simulink model "Controlador_PID_de_movimiento_discreto"  (R2023b)
settings: Solver=VariableStepAuto  StartTime=0.0  StopTime=14  RelTol=1e-3
values from neighbouring files (symbols this model uses):
  alpha_Cu = 3.9e-3    (= 0.0039)    [definicio_cte.m]
  b_a = 0.0396    [definicio_cte.m]
  b_eq = b_m + b_l/(r^2)    (= 1.98611111111e-05)    [definicio_cte.m]
  C_ts = 0.818    [definicio_cte.m]
  g = 9.80665    [definicio_cte.m]
  J_eq = J_m + J_l/(r^2)    (= 1.97847222222e-05)    [definicio_cte.m]
  k_l = m*l_cm + m_l*l_l    (= 0.25)    [definicio_cte.m]
  K_omega_2 = 3.0720e7    (= 30720000)    [definicio_cte.m]
  K_sa = 31.656    [definicio_cte.m]
  K_theta_2 = 9600    [definicio_cte.m]
  K_theta_i = 3.2768e10    (= 32768000000)    [definicio_cte.m]
  L_d = 6.6e-3    (= 0.0066)    [definicio_cte.m]
  L_ls = 0.8e-3    (= 0.0008)    [definicio_cte.m]
  L_q = 5.8e-3    (= 0.0058)    [definicio_cte.m]
  lambda_m = 0.016    [definicio_cte.m]
  lim_inf = -sqrt(2) * 48 / sqrt(3)    [definicio_cte.m]
  lim_sup = sqrt(2) * 48 / sqrt(3)    [definicio_cte.m]
  P_p = 3    [definicio_cte.m]
  r = 120    [definicio_cte.m]
  R_0 = 5000 * L_ls    (= 4)    [definicio_cte.m]
  R_d = 5000 * L_d    (= 33)    [definicio_cte.m]
  R_q = 5000 * L_q    (= 29)    [definicio_cte.m]
  R_sREF = 1.02    [definicio_cte.m]
  R_tsamb = 146.7    [definicio_cte.m]
  T_amb = 25    [definicio_cte.m]
  T_sREF = 20    [definicio_cte.m]
  tau = 20    [definicio_cte.m]
  Ts = 1.256e-4    (= 0.0001256)    [definicio_cte.m]
  w_modul = 6000*4    (= 24000)    [definicio_cte.m]
  wn_i = 6000*3    (= 18000)    [definicio_cte.m]
  wn_theta = 2000*3    (= 6000)    [definicio_cte.m]
  xita_i = 1    [definicio_cte.m]
  xita_modul = 1    [definicio_cte.m]
  xita_theta = 1    [definicio_cte.m]
undefined symbols (not defined in the file or in its folder): K_sia, magnitude
libraries: simulink x16
(part 1 of 2)
settings Model: Creator=MSI  LastModifiedBy=MSI

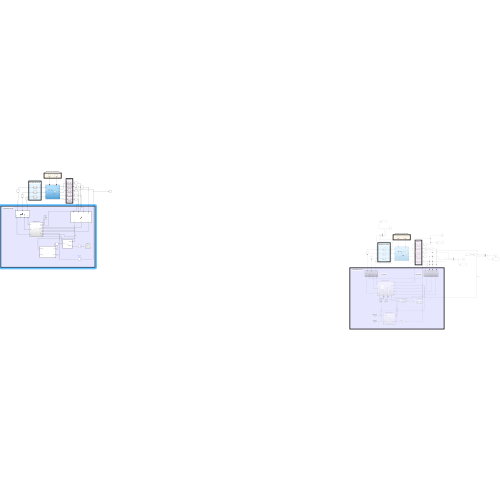
[thumbnail: Simulink's stored preview of the top-level diagram]
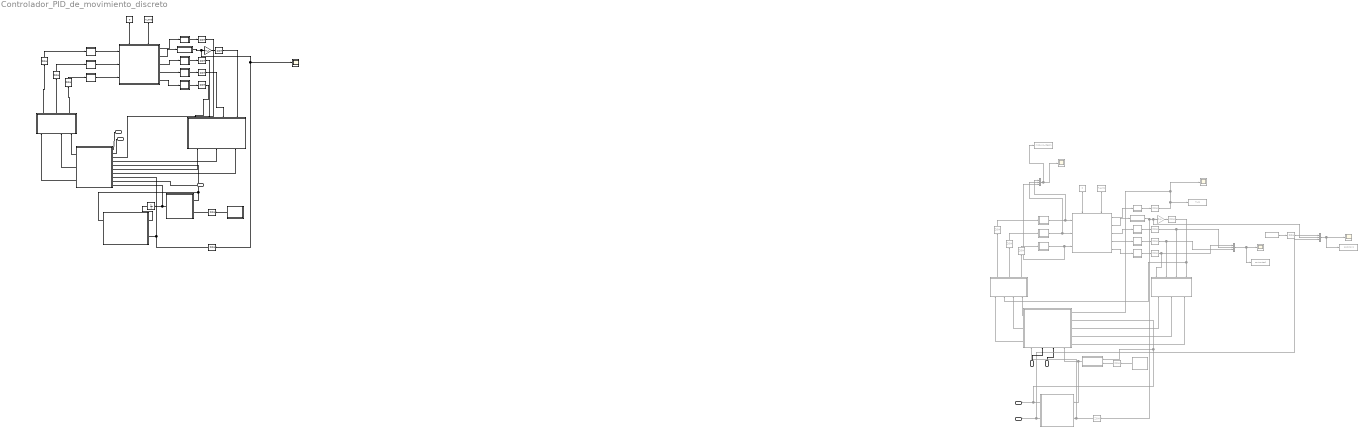
== system Controlador_PID_de_movimiento_discreto ==
  note: Controlador Parcial
  note: Sensores
  note: Entradas de perturbación
  note: Modulador de Tensión
  note: Modulador de Tensión
  note: Controlador Parcial
  note: T.P Directa
  note: Sensores
  note: Entradas de perturbación
  note: T.P Inversa
  i0s_ref : Inport
  ids_ref : Inport  Port=2
  g : Inport  Port=3
  ids*1 : Inport  Port=4
  i0s*1 : Inport  Port=5
  . : Subsystem
      settings: PortSchema="{\"entries\":[{\"content\":{\"sides\":[{\"content\":{\"connectorIds\":[\"In1\",\"In2\",\"In3\"]},\"type\":\"ConnectorPlacement.EquallySpacedRectSide\",\"uuid\":\"a2221977-a2db-4f9f-a6b6-e4e93ab83132\"},{\"content\":{\"connectorIds\":[\"Out1\",\"Out2\",\"Out3\",\"Out4\",\"Out5\"],\"side\":\"RIGHT\"},\"type\":\"ConnectorPlacement.EquallySpacedRectSide\",\"uuid\":\"4d1b64fb-cd5f-444c-9c55-dd968f667727\"},{\"content\":{\"connectorIds\":[\"In4\",\"In5\"],\"side\":\"TOP\"},\"type\":\"ConnectorPlacement.EquallySpacedRectSide\",\"uuid\":\"feec2d7e-2013-4827-9d2d-5413e6a364ce\"},{\"content\":{\"side\":\"BOTTOM\"},\"type\":\"ConnectorPlacement.EquallySpacedRectSide\",\"uuid\":\"a4e68a75-7272-4a37-88ea-97e0fe693470\"}]},\"type\":\"ConnectorPlacement.EquallySpacedConnector\",\"uuid\":\"3fef7616-1be8-4199-84fe-e5c97ae42ef2\"}],\"packageUris\":[\"http://schema.mathworks.com/mf0/Connector/R2020b\"],\"version\":\"1.0\"}"
  .1 : Subsystem  Commented=on
      settings: PortSchema="{\"entries\":[{\"content\":{\"sides\":[{\"content\":{\"connectorIds\":[\"In1\",\"In2\",\"In3\"]},\"type\":\"ConnectorPlacement.EquallySpacedRectSide\",\"uuid\":\"a2221977-a2db-4f9f-a6b6-e4e93ab83132\"},{\"content\":{\"connectorIds\":[\"Out1\",\"Out2\",\"Out3\",\"Out4\",\"Out5\"],\"side\":\"RIGHT\"},\"type\":\"ConnectorPlacement.EquallySpacedRectSide\",\"uuid\":\"4d1b64fb-cd5f-444c-9c55-dd968f667727\"},{\"content\":{\"connectorIds\":[\"In4\",\"In5\"],\"side\":\"TOP\"},\"type\":\"ConnectorPlacement.EquallySpacedRectSide\",\"uuid\":\"feec2d7e-2013-4827-9d2d-5413e6a364ce\"},{\"content\":{\"side\":\"BOTTOM\"},\"type\":\"ConnectorPlacement.EquallySpacedRectSide\",\"uuid\":\"a4e68a75-7272-4a37-88ea-97e0fe693470\"}]},\"type\":\"ConnectorPlacement.EquallySpacedConnector\",\"uuid\":\"3fef7616-1be8-4199-84fe-e5c97ae42ef2\"}],\"packageUris\":[\"http://schema.mathworks.com/mf0/Connector/R2020b\"],\"version\":\"1.0\"}"
  Constant : Constant  Value=T_amb
  Constant1 : Constant  Value=0
  Constant2 : Constant  Commented=on  Value=T_amb
  Constant3 : Constant  Commented=on  Value=0
  Controlador PID de movimiento discreto1 : Subsystem  Commented=on
  From Workspace1 : FromWorkspace  Commented=on  VariableName=theta_m_Referencia
  Gain1 : Gain  Commented=on  Gain=P_p
  Gain11 : Gain  Gain=P_p
  MATLAB Function : MATLAB Function  TreatAsAtomicUnit=on
  MATLAB Function1 : MATLAB Function  TreatAsAtomicUnit=on
  MATLAB Function2 : MATLAB Function  TreatAsAtomicUnit=on
  MATLAB Function3 : MATLAB Function  TreatAsAtomicUnit=on
  Modulador de torque : Subsystem
  Modulador de torque2 : Subsystem  Commented=on
      settings: PortSchema="{\"entries\":[{\"content\":{\"sides\":[{\"content\":{\"connectorIds\":[\"In1\",\"In2\",\"In3\",\"In4\",\"In5\"]},\"type\":\"ConnectorPlacement.EquallySpacedRectSide\",\"uuid\":\"ba876254-404b-4059-bbdb-b6055672551d\"},{\"content\":{\"connectorIds\":[\"Out1\",\"Out2\",\"Out3\"],\"side\":\"RIGHT\"},\"type\":\"ConnectorPlacement.EquallySpacedRectSide\",\"uuid\":\"d6c00e98-b252-4cfd-8c78-066fe91e4b4f\"},{\"content\":{\"side\":\"TOP\"},\"type\":\"ConnectorPlacement.EquallySpacedRectSide\",\"uuid\":\"a1ad4df6-e3d4-4e16-8862-f0d8c48039a3\"},{\"content\":{\"connectorIds\":[\"In6\",\"In7\",\"In8\",\"In9\"],\"side\":\"BOTTOM\"},\"type\":\"ConnectorPlacement.EquallySpacedRectSide\",\"uuid\":\"e932febf-7e12-4d57-82e2-13690bebd55b\"}]},\"type\":\"ConnectorPlacement.EquallySpacedConnector\",\"uuid\":\"921efeb3-6755-430d-9298-3d05b16ba3fc\"}],\"packageUris\":[\"http://schema.mathworks.com/mf0/Connector/R2020b\"],\"version\":\"1.0\"}"
  Mux3 : Mux  Commented=on  Inputs=3
  Mux4 : Mux  Commented=on  Inputs=3
  Mux5 : Mux  Commented=on  Inputs=3
  Scope : Scope
  Scope{1,5..7} (4 alike) : Scope  Commented=on
  Sensor temperatura : Subsystem
  Sensor temperatura1 : Subsystem  Commented=on
  Subsystem10 : Subsystem  Commented=on
  Subsystem3 : Subsystem
  Subsystem4 : Subsystem
  Subsystem5 : Subsystem
  Subsystem6 : Subsystem  Commented=on
  Subsystem7 : Subsystem  Commented=on
  Subsystem8 : Subsystem  Commented=on
  Subsystem9 : Subsystem  Commented=on
  To Workspace1 : ToWorkspace  Commented=on  VariableName=mod_no_ideal1  SaveFormat=Timeseries  SampleTime=-1
  To Workspace2 : ToWorkspace  Commented=on  VariableName=T_s1  SaveFormat=Timeseries  SampleTime=-1
  To Workspace3 : ToWorkspace  Commented=on  VariableName=posicion1  SaveFormat=Timeseries  SampleTime=-1
  To Workspace6 : ToWorkspace  Commented=on  VariableName=corrientes1  SaveFormat=Timeseries  SampleTime=-1
  Unit Delay : UnitDelay  SampleTime=Ts  HasFrameUpgradeWarning=on
  Zero-Order Hold{,1..7,9} (9 alike) : ZeroOrderHold  SampleTime=Ts
  Zero-Order Hold{11..20} (10 alike) : ZeroOrderHold  Commented=on  SampleTime=Ts
  Zero-Order Hold21 : ZeroOrderHold  Commented=on  SampleTime=-1
  Zero-Order Hold8 : ZeroOrderHold  SampleTime=-1
  observador de estados 1 : Subsystem  Commented=on
  omega_m*1 : Subsystem  Commented=on
  omega_m*2 : Subsystem
  sensor correinte : Subsystem
  sensor correinte1 : Subsystem
  sensor correinte2 : Subsystem
  sensor correinte3 : Subsystem  Commented=on
  sensor correinte4 : Subsystem  Commented=on
  sensor correinte5 : Subsystem  Commented=on
  sensor theta : Subsystem
  sensor theta1 : Subsystem  Commented=on
  omega_obs1 : Outport
  theta_obs1 : Outport  Port=2
  wires:
  i0s_ref/1 -> Modulador de torque/1(i0s_ref)
  ids_ref/1 -> Modulador de torque/2(ids_ref)
  Zero-Order Hold3/1 -> Modulador de torque/3(T_stator)
  MATLAB Function3/2(f_ds) -> Modulador de torque/4(i_ds)
  MATLAB Function1/1(omega_obs) -> Modulador de torque/5(omega_m), MATLAB Function/1(omega_m)
  MATLAB Function3/1(f_qs) -> Modulador de torque/6(i_qs)
  MATLAB Function3/3(f_0s) -> Modulador de torque/7(i_0s)
  g/1 -> Modulador de torque/9(g)
  MATLAB Function/1(T_m_ref) -> Unit Delay/1, Modulador de torque/10(T_m'*)
  Modulador de torque/1(V0s) -> MATLAB Function2/4(f_0s)
  Modulador de torque/2(Vds) -> MATLAB Function2/3(f_ds)
  Modulador de torque/3(Vqs) -> MATLAB Function2/1(f_qs)
  Zero-Order Hold6/1 -> MATLAB Function3/3(f_cs)
  sensor correinte1/1(y_i) -> Zero-Order Hold6/1  "ic"
  sensor theta/1(y_theta) -> Scope/1, Zero-Order Hold9/1, Gain11/1  "medida"
  Zero-Order Hold5/1 -> MATLAB Function3/2(f_bs)
  Subsystem3/1(v_a) -> ./1(v_a)  "va"
  sensor correinte/1(y_i) -> Zero-Order Hold5/1  "ib"
  ./4(i_cs) -> sensor correinte1/1(u_i)
  Constant1/1 -> ./4(T_ld)
  Subsystem5/1(v_c) -> ./3(v_c)  "vc"
  ./5(i_as) -> sensor correinte2/1(u_i)
  Zero-Order Hold/1 -> Subsystem4/1(u_a)
  ./1(T_s) -> Sensor temperatura/1(u)
  ./2(theta_m) -> sensor theta/1(u_theta)
  Zero-Order Hold4/1 -> MATLAB Function3/4(theta_r)
  Zero-Order Hold7/1 -> MATLAB Function3/1(f_as)
  Zero-Order Hold2/1 -> Subsystem5/1(u_a)
  ./3(i_bs) -> sensor correinte/1(u_i)
  Sensor temperatura/1(y) -> Zero-Order Hold3/1
  Constant/1 -> ./5(T_amb)
  Gain11/1 -> Zero-Order Hold4/1
  Subsystem4/1(v_b) -> ./2(v_b)  "vb"
  Zero-Order Hold1/1 -> Subsystem3/1(u_a)
  sensor correinte2/1(y_i) -> Zero-Order Hold7/1  "ia"
  Subsystem7/1(f_qs) -> Modulador de torque2/3(i_qs)  "i_qs"
  Subsystem7/2(f_ds) -> Modulador de torque2/4(i_ds)  "i_ds"
  i0s*1/1 -> Modulador de torque2/7(i0s*)  "i0s*"
  Subsystem8/1(v_a) -> Mux5/1, .1/1(v_a)  "va"
  sensor correinte3/1(y_i) -> Zero-Order Hold17/1  "ib"
  From Workspace1/1 -> Zero-Order Hold13/1  "referencia"
  Zero-Order Hold17/1 -> Mux4/2, Subsystem7/3(f_bs)
  Modulador de torque2/3(Vqs) -> Subsystem6/1(f_qs)
  Zero-Order Hold20/1 -> Modulador de torque2/9(theta_m), observador de estados 1/2(theta_m)  "medida"
  Mux5/1 -> To Workspace1/1, Scope7/1
  .1/4(i_cs) -> sensor correinte4/1(u_i)
  Zero-Order Hold18/1 -> Mux4/3, Subsystem7/2(f_cs)
  Zero-Order Hold21/1 -> Controlador PID de movimiento discreto1/2(omega_m*)
  omega_m*1/1(vel trapezoidal) -> Zero-Order Hold21/1
  Mux3/1 -> To Workspace3/1, Scope5/1
  observador de estados 1/2(theta_obs) -> theta_obs1/1, Mux3/3  "observada"
  ids*1/1 -> Modulador de torque2/8(ids*)  "ids*"
  Zero-Order Hold13/1 -> Mux3/1
  Zero-Order Hold11/1 -> Subsystem9/1(u_a)
  Subsystem7/3(f_0s) -> Modulador de torque2/5(i_0s)  "i_0s"
  Constant3/1 -> .1/4(T_ld)
  Controlador PID de movimiento discreto1/1(T_m'*) -> observador de estados 1/1(T_m'*), Modulador de torque2/6(T_m'*)  "T_m'*"
  Modulador de torque2/1(V0s) -> Subsystem6/4(f_0s)
  Subsystem6/3(f_cs) -> Zero-Order Hold14/1
  Subsystem10/1(v_c) -> Mux5/3, .1/3(v_c)  "vc"
  sensor correinte5/1(y_i) -> Zero-Order Hold19/1  "ia"
  .1/5(i_as) -> sensor correinte5/1(u_i)
  Constant2/1 -> .1/5(T_amb)
  Modulador de torque2/2(Vds) -> Subsystem6/3(f_ds)
  Subsystem9/1(v_b) -> Mux5/2, .1/2(v_b)  "vb"
  Gain1/1 -> Zero-Order Hold16/1
  Zero-Order Hold12/1 -> Subsystem8/1(u_a)
  .1/1(T_s) -> Sensor temperatura1/1(u)
  .1/2(theta_m) -> sensor theta1/1(u_theta)
  Sensor temperatura1/1(y) -> Zero-Order Hold15/1
  Subsystem6/2(f_bs) -> Zero-Order Hold11/1
  observador de estados 1/1(omega_obs) -> Modulador de torque2/2(omega_m), Controlador PID de movimiento discreto1/1(omega_m), omega_obs1/1
  .1/3(i_bs) -> sensor correinte3/1(u_i)
  Zero-Order Hold14/1 -> Subsystem10/1(u_a)
  Zero-Order Hold15/1 -> Modulador de torque2/1(T_s), Scope1/1, To Workspace2/1
  Mux4/1 -> To Workspace6/1, Scope6/1
  Zero-Order Hold19/1 -> Subsystem7/1(f_as), Mux4/1
  sensor correinte4/1(y_i) -> Zero-Order Hold18/1  "ic"
  sensor theta1/1(y_theta) -> Zero-Order Hold20/1, Mux3/2, Gain1/1  "medida"
  Subsystem6/1(f_as) -> Zero-Order Hold12/1
  Zero-Order Hold16/1 -> Subsystem6/2(theta_r), Subsystem7/4(theta_r)
  MATLAB Function2/3(f_cs) -> Zero-Order Hold2/1
  MATLAB Function2/2(f_bs) -> Zero-Order Hold/1
  MATLAB Function2/1(f_as) -> Zero-Order Hold1/1
  Zero-Order Hold9/1 -> Modulador de torque/8(theta_m), MATLAB Function1/2(theta_m)
  omega_m*2/1(vel trapezoidal) -> Zero-Order Hold8/1
  Zero-Order Hold8/1 -> MATLAB Function/2(omega_m_ref)
  Unit Delay/1 -> MATLAB Function1/1(T_m_ref)

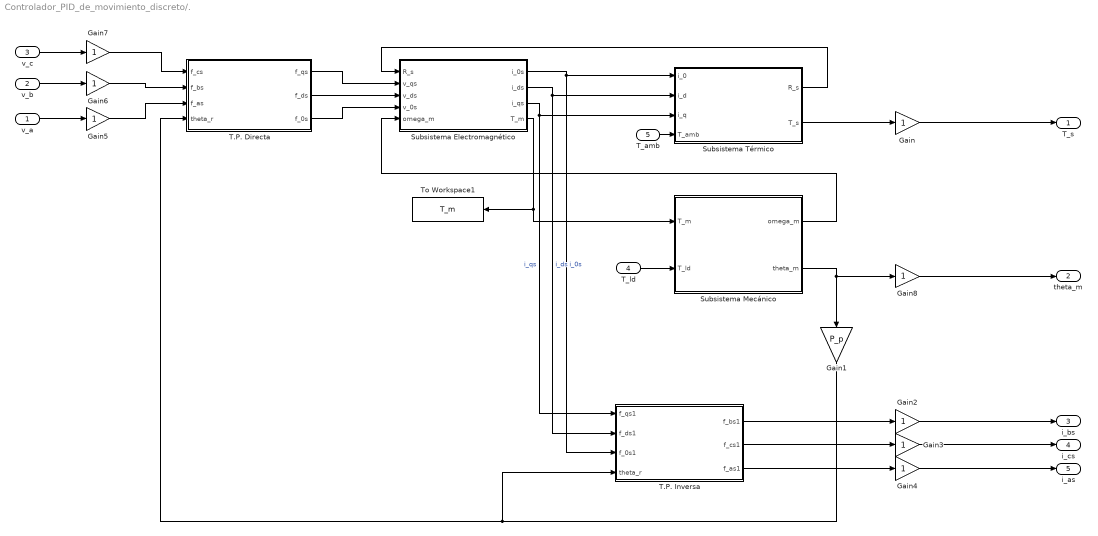
== system Controlador_PID_de_movimiento_discreto/. ==
  v_a : Inport
  v_b : Inport  Port=2
  v_c : Inport  Port=3
  T_ld : Inport  Port=4
  T_amb : Inport  Port=5
  Gain{,2..8} (8 alike) : Gain
  Gain1 : Gain  Gain=P_p
  Subsistema Electromagnético : Subsystem
  Subsistema Mecánico : Subsystem
  Subsistema Térmico : Subsystem
  T.P. Directa : Subsystem
  T.P. Inversa : Subsystem
  To Workspace1 : ToWorkspace  VariableName=T_m  SaveFormat=Timeseries  SampleTime=-1
  T_s : Outport
  theta_m : Outport  Port=2
  i_bs : Outport  Port=3
  i_cs : Outport  Port=4
  i_as : Outport  Port=5
  wires:
  Subsistema Térmico/1(R_s) -> Subsistema Electromagnético/1(R_s)
  T.P. Directa/1(f_qs) -> Subsistema Electromagnético/2(v_qs)
  T.P. Inversa/1(f_bs1) -> Gain2/1
  Subsistema Mecánico/1(omega_m) -> Subsistema Electromagnético/5(omega_m)
  Subsistema Electromagnético/1(i_0s) -> Subsistema Térmico/1(i_0), T.P. Inversa/3(f_0s1)  "i_0s"
  Subsistema Mecánico/2(theta_m) -> Gain1/1, Gain8/1
  Gain6/1 -> T.P. Directa/2(f_bs)
  Subsistema Electromagnético/4(T_m) -> Subsistema Mecánico/1(T_m), To Workspace1/1
  Gain3/1 -> i_cs/1
  Subsistema Electromagnético/2(i_ds) -> T.P. Inversa/2(f_ds1), Subsistema Térmico/2(i_d)  "i_ds"
  Gain2/1 -> i_bs/1
  T_amb/1 -> Subsistema Térmico/4(T_amb)
  v_b/1 -> Gain6/1
  v_c/1 -> Gain7/1
  v_a/1 -> Gain5/1
  Subsistema Térmico/2(T_s) -> Gain/1
  Subsistema Electromagnético/3(i_qs) -> T.P. Inversa/1(f_qs1), Subsistema Térmico/3(i_q)  "i_qs"
  Gain4/1 -> i_as/1
  T.P. Inversa/3(f_as1) -> Gain4/1
  T.P. Directa/3(f_0s) -> Subsistema Electromagnético/4(v_0s)
  T_ld/1 -> Subsistema Mecánico/2(T_ld)
  T.P. Inversa/2(f_cs1) -> Gain3/1
  Gain8/1 -> theta_m/1
  Gain7/1 -> T.P. Directa/1(f_cs)
  Gain/1 -> T_s/1
  Gain1/1 -> T.P. Directa/4(theta_r), T.P. Inversa/4(theta_r)
  T.P. Directa/2(f_ds) -> Subsistema Electromagnético/3(v_ds)
  Gain5/1 -> T.P. Directa/3(f_as)

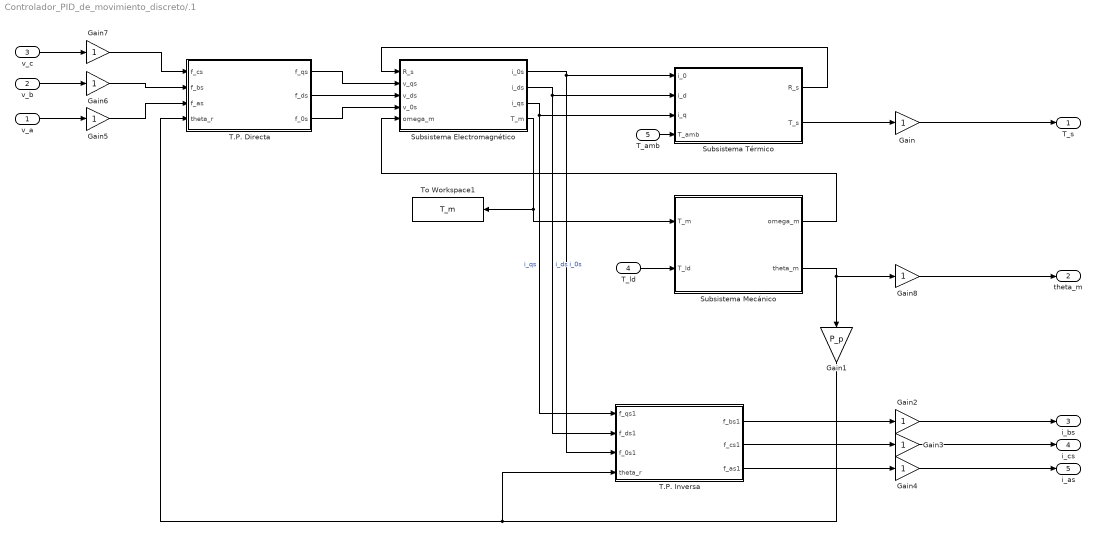
== system Controlador_PID_de_movimiento_discreto/.1 ==
  v_a : Inport
  v_b : Inport  Port=2
  v_c : Inport  Port=3
  T_ld : Inport  Port=4
  T_amb : Inport  Port=5
  Gain{,2..8} (8 alike) : Gain
  Gain1 : Gain  Gain=P_p
  Subsistema Electromagnético : Subsystem
  Subsistema Mecánico : Subsystem
  Subsistema Térmico : Subsystem
  T.P. Directa : Subsystem
  T.P. Inversa : Subsystem
  To Workspace1 : ToWorkspace  VariableName=T_m  SaveFormat=Timeseries  SampleTime=-1
  T_s : Outport
  theta_m : Outport  Port=2
  i_bs : Outport  Port=3
  i_cs : Outport  Port=4
  i_as : Outport  Port=5
  wires:
  Subsistema Térmico/1(R_s) -> Subsistema Electromagnético/1(R_s)
  T.P. Directa/1(f_qs) -> Subsistema Electromagnético/2(v_qs)
  T.P. Inversa/1(f_bs1) -> Gain2/1
  Subsistema Mecánico/1(omega_m) -> Subsistema Electromagnético/5(omega_m)
  Subsistema Electromagnético/1(i_0s) -> Subsistema Térmico/1(i_0), T.P. Inversa/3(f_0s1)  "i_0s"
  Subsistema Mecánico/2(theta_m) -> Gain1/1, Gain8/1
  Gain6/1 -> T.P. Directa/2(f_bs)
  Subsistema Electromagnético/4(T_m) -> Subsistema Mecánico/1(T_m), To Workspace1/1
  Gain3/1 -> i_cs/1
  Subsistema Electromagnético/2(i_ds) -> T.P. Inversa/2(f_ds1), Subsistema Térmico/2(i_d)  "i_ds"
  Gain2/1 -> i_bs/1
  T_amb/1 -> Subsistema Térmico/4(T_amb)
  v_b/1 -> Gain6/1
  v_c/1 -> Gain7/1
  v_a/1 -> Gain5/1
  Subsistema Térmico/2(T_s) -> Gain/1
  Subsistema Electromagnético/3(i_qs) -> T.P. Inversa/1(f_qs1), Subsistema Térmico/3(i_q)  "i_qs"
  Gain4/1 -> i_as/1
  T.P. Inversa/3(f_as1) -> Gain4/1
  T.P. Directa/3(f_0s) -> Subsistema Electromagnético/4(v_0s)
  T_ld/1 -> Subsistema Mecánico/2(T_ld)
  T.P. Inversa/2(f_cs1) -> Gain3/1
  Gain8/1 -> theta_m/1
  Gain7/1 -> T.P. Directa/1(f_cs)
  Gain/1 -> T_s/1
  Gain1/1 -> T.P. Directa/4(theta_r), T.P. Inversa/4(theta_r)
  T.P. Directa/2(f_ds) -> Subsistema Electromagnético/3(v_ds)
  Gain5/1 -> T.P. Directa/3(f_as)

== system Controlador_PID_de_movimiento_discreto/Controlador PID de movimiento discreto1 ==
  omega_m : Inport
  omega_m* : Inport  Port=2
  Gain10 : Gain  Gain=K_sa
  Gain12 : Gain  Gain=K_sia
  Gain9 : Gain  Gain=b_a
  Integrador discreto : Subsystem
  Integrador discreto1 : Subsystem
  Sum : Sum  Inputs=+++
  Sum1 : Sum  Inputs=|-+
  T_m'* : Outport
  wires:
  omega_m*/1 -> Sum1/2
  Integrador discreto1/1(y) -> Integrador discreto/1(u), Gain10/1  "e_theta"
  Gain12/1 -> Sum/1
  Integrador discreto/1(y) -> Gain12/1  "integral_e_theta"
  Sum1/1 -> Gain9/1, Integrador discreto1/1(u)  "e_omega_m"
  Sum/1 -> T_m'*/1  "T_m'*"
  Gain9/1 -> Sum/3
  Gain10/1 -> Sum/2
  omega_m/1 -> Sum1/1

== system Controlador_PID_de_movimiento_discreto/Modulador de torque ==
  i0s_ref : Inport
  ids_ref : Inport  Port=2
  T_stator : Inport  Port=3
  i_ds : Inport  Port=4
  omega_m : Inport  Port=5
  i_qs : Inport  Port=6
  i_0s : Inport  Port=7
  theta_m : Inport  Port=8
  g : Inport  Port=9
  T_m'* : Inport  Port=10
  MATLAB Function2 : MATLAB Function  TreatAsAtomicUnit=on
  MATLAB Function3 : MATLAB Function  TreatAsAtomicUnit=on
  MATLAB Function4 : MATLAB Function  TreatAsAtomicUnit=on
  V0s : Outport
  Vds : Outport  Port=2
  Vqs : Outport  Port=3
  wires:
  i_ds/1 -> MATLAB Function2/5(i_ds), MATLAB Function3/2(i_ds), MATLAB Function4/4(i_ds)
  i_0s/1 -> MATLAB Function3/3(i_0s), MATLAB Function4/5(i_0s)
  i_qs/1 -> MATLAB Function3/1(i_qs), MATLAB Function4/3(i_qs)
  MATLAB Function3/2(Vds_ref) -> MATLAB Function4/7(Vds_ref)
  omega_m/1 -> MATLAB Function2/1(omega_obs), MATLAB Function4/2(omega_m)
  MATLAB Function3/1(V0s_ref) -> MATLAB Function4/6(V0s_ref)
  T_m'*/1 -> MATLAB Function2/3(T_m_ref)
  MATLAB Function4/3(Vqs) -> Vqs/1
  i0s_ref/1 -> MATLAB Function3/6(i0s_ref)
  ids_ref/1 -> MATLAB Function3/5(ids_ref)
  theta_m/1 -> MATLAB Function2/2(theta_m)
  g/1 -> MATLAB Function2/4(g)
  MATLAB Function3/3(Vqs_ref) -> MATLAB Function4/8(Vqs_ref)
  MATLAB Function2/1(iqs_ref) -> MATLAB Function3/4(iqs_ref)
  MATLAB Function4/2(Vds) -> Vds/1
  MATLAB Function4/1(V0s) -> V0s/1
  T_stator/1 -> MATLAB Function4/1(T_stator)

== system Controlador_PID_de_movimiento_discreto/Modulador de torque2 ==
  T_s : Inport
  omega_m : Inport  Port=2
  i_qs : Inport  Port=3
  i_ds : Inport  Port=4
  i_0s : Inport  Port=5
  T_m'* : Inport  Port=6
  i0s* : Inport  Port=7
  ids* : Inport  Port=8
  theta_m : Inport  Port=9
  Constant1 : Constant  Value=g
  Desacoplamiento de retroalimentaciones fisicas naturales : Subsystem
      settings: PortSchema="{\"entries\":[{\"content\":{\"sides\":[{\"content\":{\"connectorIds\":[\"In1\",\"In2\",\"In3\",\"In4\",\"In5\"]},\"type\":\"ConnectorPlacement.EquallySpacedRectSide\",\"uuid\":\"229cb02b-d48c-446f-ba32-c62713e9b887\"},{\"content\":{\"connectorIds\":[\"Out1\",\"Out2\",\"Out3\"],\"side\":\"RIGHT\"},\"type\":\"ConnectorPlacement.EquallySpacedRectSide\",\"uuid\":\"d1560b4a-f0ce-405c-b2ec-43a69c5457bd\"},{\"content\":{\"side\":\"TOP\"},\"type\":\"ConnectorPlacement.EquallySpacedRectSide\",\"uuid\":\"c93a9a8d-95cd-44a7-8de3-b4ab0da15153\"},{\"content\":{\"connectorIds\":[\"In6\",\"In7\",\"In8\"],\"side\":\"BOTTOM\"},\"type\":\"ConnectorPlacement.EquallySpacedRectSide\",\"uuid\":\"61b8912b-c246-41e9-a841-420011d131cc\"}]},\"type\":\"ConnectorPlacement.EquallySpacedConnector\",\"uuid\":\"53c75e92-39e8-4743-a399-9153728077fe\"}],\"packageUris\":[\"http://schema.mathworks.com/mf0/Connector/R2020b\"],\"version\":\"1.0\"}"
  Lazo de corriente : Subsystem
      settings: PortSchema="{\"entries\":[{\"content\":{\"sides\":[{\"content\":{\"connectorIds\":[\"In1\",\"In2\",\"In3\",\"In4\"]},\"type\":\"ConnectorPlacement.EquallySpacedRectSide\",\"uuid\":\"e4a1f591-de4c-4bed-9730-a0bdcd595dfe\"},{\"content\":{\"connectorIds\":[\"Out1\",\"Out2\",\"Out3\"],\"side\":\"RIGHT\"},\"type\":\"ConnectorPlacement.EquallySpacedRectSide\",\"uuid\":\"b5219b6b-3019-4355-bcfd-890ee0fb4c54\"},{\"content\":{\"side\":\"TOP\"},\"type\":\"ConnectorPlacement.EquallySpacedRectSide\",\"uuid\":\"3e4154c5-0bb5-4a69-ba55-234c7bde9140\"},{\"content\":{\"connectorIds\":[\"In5\",\"In6\"],\"side\":\"BOTTOM\"},\"type\":\"ConnectorPlacement.EquallySpacedRectSide\",\"uuid\":\"43784307-e678-4ce2-8a7d-2ff65f16c696\"}]},\"type\":\"ConnectorPlacement.EquallySpacedConnector\",\"uuid\":\"60b6d0d3-75d2-4869-ad7d-030d7c987d05\"}],\"packageUris\":[\"http://schema.mathworks.com/mf0/Connector/R2020b\"],\"version\":\"1.0\"}"
  Lazo de torque : Subsystem
  V0s : Outport
  Vds : Outport  Port=2
  Vqs : Outport  Port=3
  wires:
  Lazo de corriente/1(V0s*) -> Desacoplamiento de retroalimentaciones fisicas naturales/6(V0s*)
  ids*/1 -> Lazo de corriente/5(ids*)
  Lazo de corriente/2(Vds*) -> Desacoplamiento de retroalimentaciones fisicas naturales/7(Vds*)
  i0s*/1 -> Lazo de corriente/6(i0s*)
  i_ds/1 -> Desacoplamiento de retroalimentaciones fisicas naturales/4(i_ds), Lazo de corriente/2(i_ds), Lazo de torque/4(i_ds)
  i_0s/1 -> Lazo de corriente/3(i_0s), Desacoplamiento de retroalimentaciones fisicas naturales/5(i_0s)
  omega_m/1 -> Desacoplamiento de retroalimentaciones fisicas naturales/2(omega_m), Lazo de torque/1(omega_m)
  Lazo de corriente/3(Vqs*) -> Desacoplamiento de retroalimentaciones fisicas naturales/8(Vqs*)
  i_qs/1 -> Lazo de corriente/1(i_qs), Desacoplamiento de retroalimentaciones fisicas naturales/3(i_qs)
  Desacoplamiento de retroalimentaciones fisicas naturales/1(Vqs) -> Vqs/1
  Desacoplamiento de retroalimentaciones fisicas naturales/3(V0s) -> V0s/1
  Constant1/1 -> Lazo de torque/3(g)  "g"
  Lazo de torque/1(iqs*) -> Lazo de corriente/4(iqs*)
  T_m'*/1 -> Lazo de torque/2(T_m'*)
  Desacoplamiento de retroalimentaciones fisicas naturales/2(Vds) -> Vds/1
  T_s/1 -> Desacoplamiento de retroalimentaciones fisicas naturales/1(T_s)
  theta_m/1 -> Lazo de torque/5(theta_m)

== system Controlador_PID_de_movimiento_discreto/Sensor temperatura ==
  u : Inport
  Gain9 : Gain  Gain=1/tau
  Integrator : Integrator  InitialCondition=T_amb
  Sum : Sum  Inputs=|+-
  y : Outport
  wires:
  Integrator/1 -> y/1, Sum/2
  u/1 -> Sum/1
  Sum/1 -> Gain9/1
  Gain9/1 -> Integrator/1

== system Controlador_PID_de_movimiento_discreto/Sensor temperatura1 ==
  u : Inport
  Gain9 : Gain  Gain=1/tau
  Integrator : Integrator  InitialCondition=T_amb
  Sum : Sum  Inputs=|+-
  y : Outport
  wires:
  Integrator/1 -> y/1, Sum/2
  u/1 -> Sum/1
  Sum/1 -> Gain9/1
  Gain9/1 -> Integrator/1

== system Controlador_PID_de_movimiento_discreto/Subsystem10 ==
  u_a : Inport
  Saturation : Saturate  UpperLimit=lim_sup  LowerLimit=lim_inf
  Subsystem : Subsystem
  v_c : Outport
  wires:
  u_a/1 -> Subsystem/1(u_a)
  Subsystem/1(y_a) -> Saturation/1
  Saturation/1 -> v_c/1

== system Controlador_PID_de_movimiento_discreto/Subsystem3 ==
  u_a : Inport
  Saturation : Saturate  UpperLimit=lim_sup  LowerLimit=lim_inf
  Subsystem : Subsystem
  v_a : Outport
  wires:
  u_a/1 -> Subsystem/1(u_a)
  Subsystem/1(y_a) -> Saturation/1
  Saturation/1 -> v_a/1

== system Controlador_PID_de_movimiento_discreto/Subsystem4 ==
  u_a : Inport
  Saturation : Saturate  UpperLimit=lim_sup  LowerLimit=lim_inf
  Subsystem : Subsystem
  v_b : Outport
  wires:
  Saturation/1 -> v_b/1
  Subsystem/1(y_a) -> Saturation/1
  u_a/1 -> Subsystem/1(u_a)

== system Controlador_PID_de_movimiento_discreto/Subsystem5 ==
  u_a : Inport
  Saturation : Saturate  UpperLimit=lim_sup  LowerLimit=lim_inf
  Subsystem : Subsystem
  v_c : Outport
  wires:
  u_a/1 -> Subsystem/1(u_a)
  Subsystem/1(y_a) -> Saturation/1
  Saturation/1 -> v_c/1

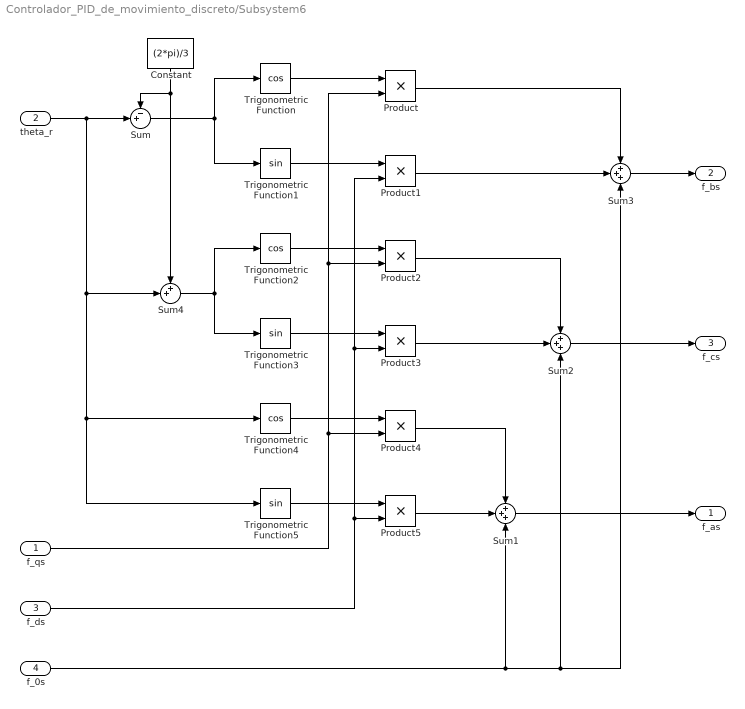
== system Controlador_PID_de_movimiento_discreto/Subsystem6 ==
  f_qs : Inport
  theta_r : Inport  Port=2
  f_ds : Inport  Port=3
  f_0s : Inport  Port=4
  Constant : Constant  Value=(2*pi)/3
  Product{,1..5} (6 alike) : Product
  Sum : Sum  Inputs=-+|
  Sum1 : Sum  Inputs=+++
  Sum2 : Sum  Inputs=+++
  Sum3 : Sum  Inputs=+++
  Sum4 : Sum  Inputs=++|
  Trigonometric Function : Trigonometry  Operator=cos
  Trigonometric Function1 : Trigonometry
  Trigonometric Function2 : Trigonometry  Operator=cos
  Trigonometric Function3 : Trigonometry
  Trigonometric Function4 : Trigonometry  Operator=cos
  Trigonometric Function5 : Trigonometry
  f_as : Outport
  f_bs : Outport  Port=2
  f_cs : Outport  Port=3
  wires:
  Sum1/1 -> f_as/1
  Product5/1 -> Sum1/2
  Sum2/1 -> f_cs/1
  Product1/1 -> Sum3/2
  Trigonometric Function5/1 -> Product5/1
  Sum/1 -> Trigonometric Function1/1, Trigonometric Function/1
  Product2/1 -> Sum2/1
  Product4/1 -> Sum1/1
  f_qs/1 -> Product4/2, Product2/2, Product/2
  Product/1 -> Sum3/1
  f_0s/1 -> Sum3/3, Sum2/3, Sum1/3
  Trigonometric Function4/1 -> Product4/1
  Constant/1 -> Sum4/1, Sum/1
  Trigonometric Function2/1 -> Product2/1
  f_ds/1 -> Product5/2, Product3/2, Product1/2
  Trigonometric Function3/1 -> Product3/1
  Trigonometric Function1/1 -> Product1/1
  Sum4/1 -> Trigonometric Function3/1, Trigonometric Function2/1
  Sum3/1 -> f_bs/1
  theta_r/1 -> Sum4/2, Trigonometric Function5/1, Trigonometric Function4/1, Sum/2
  Product3/1 -> Sum2/2
  Trigonometric Function/1 -> Product/1

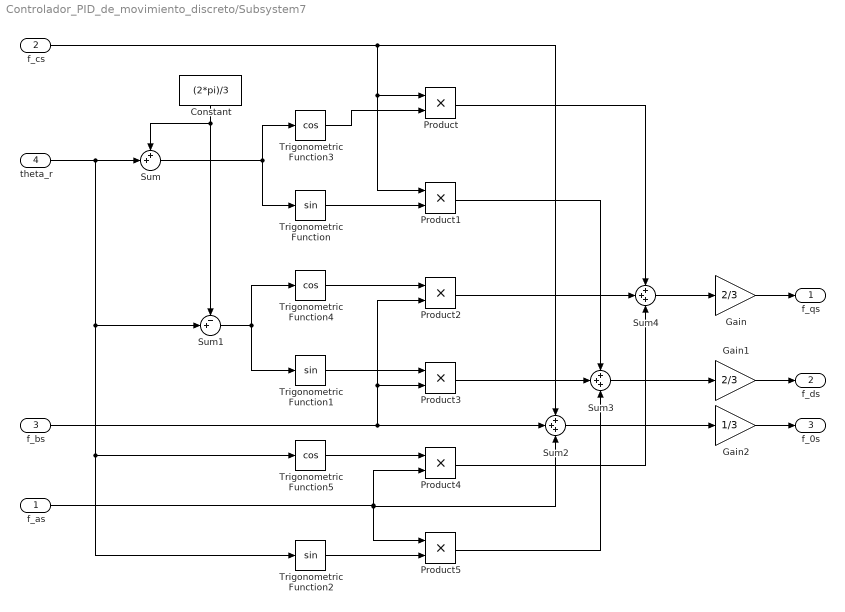
== system Controlador_PID_de_movimiento_discreto/Subsystem7 ==
  f_as : Inport
  f_cs : Inport  Port=2
  f_bs : Inport  Port=3
  theta_r : Inport  Port=4
  Constant : Constant  Value=(2*pi)/3
  Gain : Gain  Gain=2/3
  Gain1 : Gain  Gain=2/3
  Gain2 : Gain  Gain=1/3
  Product{,1..5} (6 alike) : Product
  Sum : Sum  Inputs=++|
  Sum1 : Sum  Inputs=-+|
  Sum2 : Sum  Inputs=+++
  Sum3 : Sum  Inputs=+++
  Sum4 : Sum  Inputs=+++
  Trigonometric Function : Trigonometry
  Trigonometric Function1 : Trigonometry
  Trigonometric Function2 : Trigonometry
  Trigonometric Function3 : Trigonometry  Operator=cos
  Trigonometric Function4 : Trigonometry  Operator=cos
  Trigonometric Function5 : Trigonometry  Operator=cos
  f_qs : Outport
  f_ds : Outport  Port=2
  f_0s : Outport  Port=3
  wires:
  f_cs/1 -> Product/1, Product1/1, Sum2/1
  Product3/1 -> Sum3/2
  Trigonometric Function5/1 -> Product4/1
  Constant/1 -> Sum/1, Sum1/1
  Sum1/1 -> Trigonometric Function1/1, Trigonometric Function4/1
  Gain2/1 -> f_0s/1
  Gain1/1 -> f_ds/1
  theta_r/1 -> Sum1/2, Trigonometric Function2/1, Trigonometric Function5/1, Sum/2
  Sum4/1 -> Gain/1
  Trigonometric Function1/1 -> Product3/1
  f_bs/1 -> Product2/2, Product3/2, Sum2/2
  Product4/1 -> Sum4/3
  Gain/1 -> f_qs/1
  Product/1 -> Sum4/1
  f_as/1 -> Sum2/3, Product5/1, Product4/2
  Sum2/1 -> Gain2/1
  Product2/1 -> Sum4/2
  Trigonometric Function2/1 -> Product5/2
  Sum3/1 -> Gain1/1
  Trigonometric Function/1 -> Product1/2
  Trigonometric Function3/1 -> Product/2
  Trigonometric Function4/1 -> Product2/1
  Product5/1 -> Sum3/3
  Product1/1 -> Sum3/1
  Sum/1 -> Trigonometric Function3/1, Trigonometric Function/1

== system Controlador_PID_de_movimiento_discreto/Subsystem8 ==
  u_a : Inport
  Saturation : Saturate  UpperLimit=lim_sup  LowerLimit=lim_inf
  Subsystem : Subsystem
  v_a : Outport
  wires:
  u_a/1 -> Subsystem/1(u_a)
  Subsystem/1(y_a) -> Saturation/1
  Saturation/1 -> v_a/1

== system Controlador_PID_de_movimiento_discreto/Subsystem9 ==
  u_a : Inport
  Saturation : Saturate  UpperLimit=lim_sup  LowerLimit=lim_inf
  Subsystem : Subsystem
  v_b : Outport
  wires:
  Saturation/1 -> v_b/1
  Subsystem/1(y_a) -> Saturation/1
  u_a/1 -> Subsystem/1(u_a)

== system Controlador_PID_de_movimiento_discreto/observador de estados 1 ==
  T_m'* : Inport
  theta_m : Inport  Port=2
  Gain : Gain  Gain=K_theta_i
  Gain10 : Gain  Gain=K_omega_2
  Gain12 : Gain  Gain=K_theta_2
  Gain9 : Gain  Gain=1/J_eq
  Integrador discreto : Subsystem
  Integrador discreto1 : Subsystem
  Integrador discreto2 : Subsystem
  Sum : Sum  Inputs=++|
  Sum2 : Sum  Inputs=++|
  Sum5 : Sum  Inputs=+-
  Sum6 : Sum  Inputs=++|
  omega_obs : Outport
  theta_obs : Outport  Port=2
  wires:
  Sum2/1 -> Sum/2
  Gain9/1 -> Sum2/2
  Sum/1 -> Integrador discreto1/1(u)  "domega_obs"
  theta_m/1 -> Sum5/1  "theta_m"
  T_m'*/1 -> Gain9/1
  Integrador discreto1/1(y) -> Sum6/2  "omega_obs"
  Sum6/1 -> omega_obs/1, Integrador discreto2/1(u)  "dtheta_obs"
  Gain12/1 -> Sum6/1
  Integrador discreto2/1(y) -> theta_obs/1, Sum5/2  "theta_obs"
  Gain10/1 -> Sum/1
  Gain/1 -> Integrador discreto/1(u)  "dv"
  Sum5/1 -> Gain12/1, Gain10/1, Gain/1  "e_obs_theta"
  Integrador discreto/1(y) -> Sum2/1  "v"

== system Controlador_PID_de_movimiento_discreto/omega_m*1 ==
  Ramp : simulink/Sources/Ramp  slope=1500  start=1  InitialOutput=0
  Ramp1 : simulink/Sources/Ramp  slope=-1500  start=1.1  InitialOutput=0
  Ramp2 : simulink/Sources/Ramp  slope=-1500  start=5.9  InitialOutput=0
  Ramp3 : simulink/Sources/Ramp  slope=-1500  start=8  InitialOutput=0
  Ramp4 : simulink/Sources/Ramp  slope=1500  start=6  InitialOutput=0
  Ramp5 : simulink/Sources/Ramp  slope=1500  start=8.1  InitialOutput=0
  Ramp6 : simulink/Sources/Ramp  slope=1500  start=12.9  InitialOutput=0
  Ramp7 : simulink/Sources/Ramp  slope=-1500  start=13  InitialOutput=0
  Sum1 : Sum  Inputs=++++++++
  vel trapezoidal : Outport
  wires:
  Ramp4/1 -> Sum1/4
  Ramp2/1 -> Sum1/3
  Ramp3/1 -> Sum1/5
  Ramp1/1 -> Sum1/2
  Ramp6/1 -> Sum1/7
  Ramp/1 -> Sum1/1
  Ramp5/1 -> Sum1/6
  Sum1/1 -> vel trapezoidal/1  "cuadrada"
  Ramp7/1 -> Sum1/8

== system Controlador_PID_de_movimiento_discreto/omega_m*2 ==
  Ramp : simulink/Sources/Ramp  slope=1500  start=1  InitialOutput=0
  Ramp1 : simulink/Sources/Ramp  slope=-1500  start=1.1  InitialOutput=0
  Ramp2 : simulink/Sources/Ramp  slope=-1500  start=5.9  InitialOutput=0
  Ramp3 : simulink/Sources/Ramp  slope=-1500  start=8  InitialOutput=0
  Ramp4 : simulink/Sources/Ramp  slope=1500  start=6  InitialOutput=0
  Ramp5 : simulink/Sources/Ramp  slope=1500  start=8.1  InitialOutput=0
  Ramp6 : simulink/Sources/Ramp  slope=1500  start=12.9  InitialOutput=0
  Ramp7 : simulink/Sources/Ramp  slope=-1500  start=13  InitialOutput=0
  Sum1 : Sum  Inputs=++++++++
  vel trapezoidal : Outport
  wires:
  Ramp4/1 -> Sum1/4
  Ramp2/1 -> Sum1/3
  Ramp3/1 -> Sum1/5
  Ramp1/1 -> Sum1/2
  Ramp6/1 -> Sum1/7
  Ramp/1 -> Sum1/1
  Ramp5/1 -> Sum1/6
  Sum1/1 -> vel trapezoidal/1  "cuadrada"
  Ramp7/1 -> Sum1/8

== system Controlador_PID_de_movimiento_discreto/sensor correinte ==
  u_i : Inport
  Gain10 : Gain  Gain=wn_i
  Gain12 : Gain  Gain=xita_i
  Gain13 : Gain  Gain=2
  Gain14 : Gain  Gain=(wn_i)^2
  Gain9 : Gain  Gain=(wn_i)^2
  Integrator : Integrator
  Integrator1 : Integrator
  Sum : Sum  Inputs=+--
  y_i : Outport
  wires:
  Gain12/1 -> Gain13/1
  u_i/1 -> Gain9/1
  Gain10/1 -> Gain12/1
  Gain13/1 -> Sum/3
  Integrator1/1 -> y_i/1, Gain14/1  "x_1 = y"
  Sum/1 -> Integrator/1  "y' = x_2'"
  Gain14/1 -> Sum/2
  Integrator/1 -> Gain10/1, Integrator1/1  "x_2 = x_1'"
  Gain9/1 -> Sum/1

== system Controlador_PID_de_movimiento_discreto/sensor correinte1 ==
  u_i : Inport
  Gain10 : Gain  Gain=wn_i
  Gain12 : Gain  Gain=xita_i
  Gain13 : Gain  Gain=2
  Gain14 : Gain  Gain=(wn_i)^2
  Gain9 : Gain  Gain=(wn_i)^2
  Integrator : Integrator
  Integrator1 : Integrator
  Sum : Sum  Inputs=+--
  y_i : Outport
  wires:
  Gain9/1 -> Sum/1
  Integrator/1 -> Integrator1/1, Gain10/1  "x_2 = x_1'"
  Gain14/1 -> Sum/2
  Sum/1 -> Integrator/1  "y' = x_2'"
  Integrator1/1 -> Gain14/1, y_i/1  "x_1 = y"
  Gain13/1 -> Sum/3
  Gain10/1 -> Gain12/1
  u_i/1 -> Gain9/1
  Gain12/1 -> Gain13/1

== system Controlador_PID_de_movimiento_discreto/sensor correinte2 ==
  u_i : Inport
  Gain10 : Gain  Gain=wn_i
  Gain12 : Gain  Gain=xita_i
  Gain13 : Gain  Gain=2
  Gain14 : Gain  Gain=(wn_i)^2
  Gain9 : Gain  Gain=(wn_i)^2
  Integrator : Integrator
  Integrator1 : Integrator
  Sum : Sum  Inputs=+--
  y_i : Outport
  wires:
  Gain12/1 -> Gain13/1
  u_i/1 -> Gain9/1
  Gain10/1 -> Gain12/1
  Gain13/1 -> Sum/3
  Integrator1/1 -> y_i/1, Gain14/1  "x_1 = y"
  Sum/1 -> Integrator/1  "y' = x_2'"
  Gain14/1 -> Sum/2
  Integrator/1 -> Gain10/1, Integrator1/1  "x_2 = x_1'"
  Gain9/1 -> Sum/1

== system Controlador_PID_de_movimiento_discreto/sensor correinte3 ==
  u_i : Inport
  Gain10 : Gain  Gain=wn_i
  Gain12 : Gain  Gain=xita_i
  Gain13 : Gain  Gain=2
  Gain14 : Gain  Gain=(wn_i)^2
  Gain9 : Gain  Gain=(wn_i)^2
  Integrator : Integrator
  Integrator1 : Integrator
  Sum : Sum  Inputs=+--
  y_i : Outport
  wires:
  Gain12/1 -> Gain13/1
  u_i/1 -> Gain9/1
  Gain10/1 -> Gain12/1
  Gain13/1 -> Sum/3
  Integrator1/1 -> y_i/1, Gain14/1  "x_1 = y"
  Sum/1 -> Integrator/1  "y' = x_2'"
  Gain14/1 -> Sum/2
  Integrator/1 -> Gain10/1, Integrator1/1  "x_2 = x_1'"
  Gain9/1 -> Sum/1

== system Controlador_PID_de_movimiento_discreto/sensor correinte4 ==
  u_i : Inport
  Gain10 : Gain  Gain=wn_i
  Gain12 : Gain  Gain=xita_i
  Gain13 : Gain  Gain=2
  Gain14 : Gain  Gain=(wn_i)^2
  Gain9 : Gain  Gain=(wn_i)^2
  Integrator : Integrator
  Integrator1 : Integrator
  Sum : Sum  Inputs=+--
  y_i : Outport
  wires:
  Gain9/1 -> Sum/1
  Integrator/1 -> Integrator1/1, Gain10/1  "x_2 = x_1'"
  Gain14/1 -> Sum/2
  Sum/1 -> Integrator/1  "y' = x_2'"
  Integrator1/1 -> Gain14/1, y_i/1  "x_1 = y"
  Gain13/1 -> Sum/3
  Gain10/1 -> Gain12/1
  u_i/1 -> Gain9/1
  Gain12/1 -> Gain13/1

== system Controlador_PID_de_movimiento_discreto/sensor correinte5 ==
  u_i : Inport
  Gain10 : Gain  Gain=wn_i
  Gain12 : Gain  Gain=xita_i
  Gain13 : Gain  Gain=2
  Gain14 : Gain  Gain=(wn_i)^2
  Gain9 : Gain  Gain=(wn_i)^2
  Integrator : Integrator
  Integrator1 : Integrator
  Sum : Sum  Inputs=+--
  y_i : Outport
  wires:
  Gain12/1 -> Gain13/1
  u_i/1 -> Gain9/1
  Gain10/1 -> Gain12/1
  Gain13/1 -> Sum/3
  Integrator1/1 -> y_i/1, Gain14/1  "x_1 = y"
  Sum/1 -> Integrator/1  "y' = x_2'"
  Gain14/1 -> Sum/2
  Integrator/1 -> Gain10/1, Integrator1/1  "x_2 = x_1'"
  Gain9/1 -> Sum/1

== system Controlador_PID_de_movimiento_discreto/sensor theta ==
  u_theta : Inport
  Gain10 : Gain  Gain=wn_theta
  Gain12 : Gain  Gain=xita_theta
  Gain13 : Gain  Gain=2
  Gain14 : Gain  Gain=(wn_theta)^2
  Gain9 : Gain  Gain=(wn_theta)^2
  Integrator : Integrator
  Integrator1 : Integrator
  Sum : Sum  Inputs=+--
  y_theta : Outport
  wires:
  u_theta/1 -> Gain9/1
  Gain14/1 -> Sum/2
  Gain12/1 -> Gain13/1
  Sum/1 -> Integrator/1  "y' = x_2'"
  Integrator1/1 -> y_theta/1, Gain14/1  "x_1 = y"
  Gain13/1 -> Sum/3
  Gain9/1 -> Sum/1
  Gain10/1 -> Gain12/1
  Integrator/1 -> Gain10/1, Integrator1/1  "x_2 = x_1'"

== system Controlador_PID_de_movimiento_discreto/sensor theta1 ==
  u_theta : Inport
  Gain10 : Gain  Gain=wn_theta
  Gain12 : Gain  Gain=xita_theta
  Gain13 : Gain  Gain=2
  Gain14 : Gain  Gain=(wn_theta)^2
  Gain9 : Gain  Gain=(wn_theta)^2
  Integrator : Integrator
  Integrator1 : Integrator
  Sum : Sum  Inputs=+--
  y_theta : Outport
  wires:
  u_theta/1 -> Gain9/1
  Gain14/1 -> Sum/2
  Gain12/1 -> Gain13/1
  Sum/1 -> Integrator/1  "y' = x_2'"
  Integrator1/1 -> y_theta/1, Gain14/1  "x_1 = y"
  Gain13/1 -> Sum/3
  Gain9/1 -> Sum/1
  Gain10/1 -> Gain12/1
  Integrator/1 -> Gain10/1, Integrator1/1  "x_2 = x_1'"

== system Controlador_PID_de_movimiento_discreto/./Subsistema Electromagnético ==
  R_s : Inport
  v_qs : Inport  Port=2
  v_ds : Inport  Port=3
  v_0s : Inport  Port=4
  omega_m : Inport  Port=5
  corriente_i_0s : Subsystem
  corriente_i_ds : Subsystem
  corriente_i_qs : Subsystem
  torque_T_m : Subsystem
  i_0s : Outport
  i_ds : Outport  Port=2
  i_qs : Outport  Port=3
  T_m : Outport  Port=4
  wires:
  R_s/1 -> corriente_i_qs/3(R_s), corriente_i_ds/4(R_s), corriente_i_0s/2(R_s)
  corriente_i_0s/1(i_0s) -> i_0s/1
  corriente_i_qs/1(i_qs) -> i_qs/1, torque_T_m/2(i_qs), corriente_i_ds/2(i_qs)
  corriente_i_ds/1(i_ds) -> corriente_i_qs/4(i_ds), torque_T_m/1(i_ds), i_ds/1
  v_0s/1 -> corriente_i_0s/1(v_0s)
  v_ds/1 -> corriente_i_ds/1(v_ds)
  omega_m/1 -> corriente_i_qs/1(omega_m), corriente_i_ds/3(omega_m)
  v_qs/1 -> corriente_i_qs/2(v_qs)
  torque_T_m/1(T_m) -> T_m/1

== system Controlador_PID_de_movimiento_discreto/./Subsistema Mecánico ==
  T_m : Inport
  T_ld : Inport  Port=2
  Constant : Constant  Value=g
  Gain : Gain  Gain=1/J_eq
  Gain1 : Gain  Gain=b_eq
  Gain2 : Gain  Gain=1/r
  Gain3 : Gain  Gain=k_l
  Gain4 : Gain  Gain=1/r
  Product : Product
  Sum : Sum  Inputs=-+-
  Sum1 : Sum
  Trigonometric Function : Trigonometry
  "omega_m(0) = 0\t" : Integrator
  theta_m(0) = 0 : Integrator
  omega_m : Outport
  theta_m : Outport  Port=2
  wires:
  Product/1 -> Sum1/2
  Constant/1 -> Product/1
  T_m/1 -> Sum/2
  Gain3/1 -> Product/2
  T_ld/1 -> Sum1/1
  Gain1/1 -> Sum/3
  Gain4/1 -> Sum/1
  Sum1/1 -> Gain4/1  "T_l"
  theta_m(0) = 0/1 -> Gain2/1, theta_m/1  "theta_m(t)"
  Trigonometric Function/1 -> Gain3/1
  Sum/1 -> Gain/1
  Gain2/1 -> Trigonometric Function/1
  "omega_m(0) = 0\t"/1 -> theta_m(0) = 0/1, omega_m/1, Gain1/1  "omega_m(t)"
  Gain/1 -> "omega_m(0) = 0\t"/1  "domega_m(t)/dt"

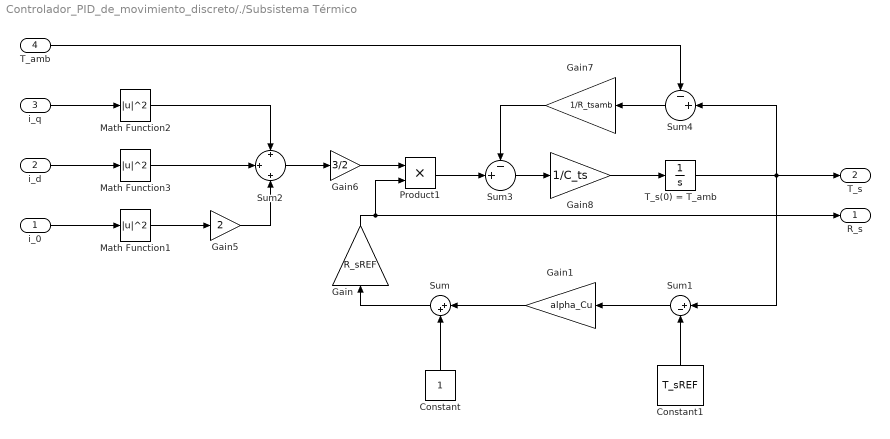
== system Controlador_PID_de_movimiento_discreto/./Subsistema Térmico ==
  i_0 : Inport
  i_d : Inport  Port=2
  i_q : Inport  Port=3
  T_amb : Inport  Port=4
  Constant : Constant
  Constant1 : Constant  Value=T_sREF
  Gain : Gain  Gain=R_sREF
  Gain1 : Gain  Gain=alpha_Cu
  Gain5 : Gain  Gain=2
  Gain6 : Gain  Gain=3/2
  Gain7 : Gain  Gain=1/R_tsamb
  Gain8 : Gain  Gain=1/C_ts
  Math Function1 : Math  Operator=magnitude^2  OutputSignalType=real
  Math Function2 : Math  Operator=magnitude^2  OutputSignalType=real
  Math Function3 : Math  Operator=magnitude^2  OutputSignalType=real
  Product1 : Product
  Sum : Sum  Inputs=|++
  Sum1 : Sum  Inputs=|+-
  Sum2 : Sum  Inputs=+|+|+
  Sum3 : Sum  Inputs=-+|
  Sum4 : Sum  Inputs=-+|
  T_s(0) = T_amb : Integrator  InitialCondition=T_amb
  R_s : Outport
  T_s : Outport  Port=2
  wires:
  i_q/1 -> Math Function2/1
  i_d/1 -> Math Function3/1
  i_0/1 -> Math Function1/1
  Gain1/1 -> Sum/1
  Gain8/1 -> T_s(0) = T_amb/1
  Sum3/1 -> Gain8/1
  Constant/1 -> Sum/2
  Product1/1 -> Sum3/2
  Sum/1 -> Gain/1
  T_amb/1 -> Sum4/1
  Math Function1/1 -> Gain5/1
  Sum4/1 -> Gain7/1
  T_s(0) = T_amb/1 -> Sum1/1, Sum4/2, T_s/1
  Sum2/1 -> Gain6/1
  Sum1/1 -> Gain1/1
  Gain6/1 -> Product1/1
  Constant1/1 -> Sum1/2
  Gain5/1 -> Sum2/3
  Gain7/1 -> Sum3/1
  Math Function2/1 -> Sum2/1
  Math Function3/1 -> Sum2/2
  Gain/1 -> R_s/1, Product1/2

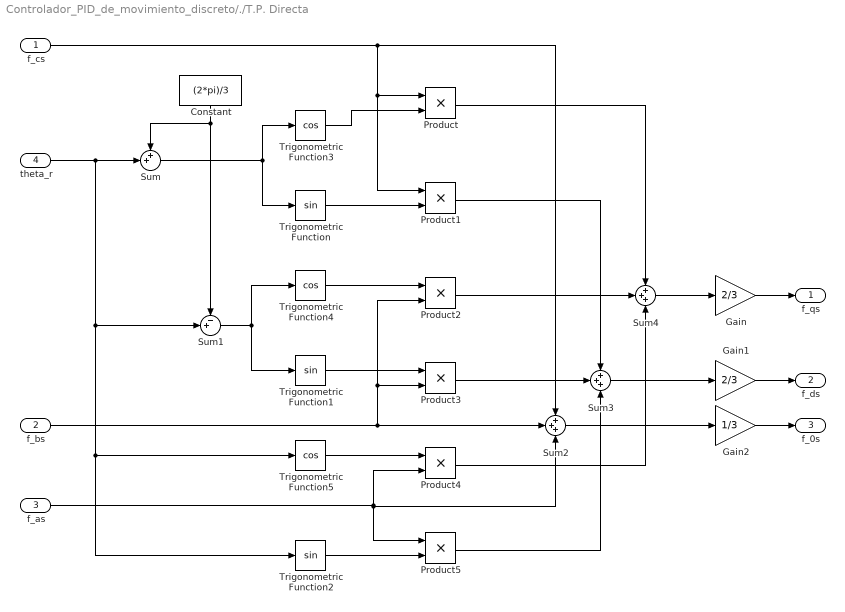
== system Controlador_PID_de_movimiento_discreto/./T.P. Directa ==
  f_cs : Inport
  f_bs : Inport  Port=2
  f_as : Inport  Port=3
  theta_r : Inport  Port=4
  Constant : Constant  Value=(2*pi)/3
  Gain : Gain  Gain=2/3
  Gain1 : Gain  Gain=2/3
  Gain2 : Gain  Gain=1/3
  Product{,1..5} (6 alike) : Product
  Sum : Sum  Inputs=++|
  Sum1 : Sum  Inputs=-+|
  Sum2 : Sum  Inputs=+++
  Sum3 : Sum  Inputs=+++
  Sum4 : Sum  Inputs=+++
  Trigonometric Function : Trigonometry
  Trigonometric Function1 : Trigonometry
  Trigonometric Function2 : Trigonometry
  Trigonometric Function3 : Trigonometry  Operator=cos
  Trigonometric Function4 : Trigonometry  Operator=cos
  Trigonometric Function5 : Trigonometry  Operator=cos
  f_qs : Outport
  f_ds : Outport  Port=2
  f_0s : Outport  Port=3
  wires:
  Product5/1 -> Sum3/3
  theta_r/1 -> Sum1/2, Trigonometric Function2/1, Trigonometric Function5/1, Sum/2
  f_bs/1 -> Product2/2, Product3/2, Sum2/2
  f_cs/1 -> Product/1, Product1/1, Sum2/1
  Trigonometric Function5/1 -> Product4/1
  Sum1/1 -> Trigonometric Function1/1, Trigonometric Function4/1
  Constant/1 -> Sum/1, Sum1/1
  Sum/1 -> Trigonometric Function3/1, Trigonometric Function/1
  f_as/1 -> Sum2/3, Product5/1, Product4/2
  Gain2/1 -> f_0s/1
  Trigonometric Function2/1 -> Product5/2
  Trigonometric Function1/1 -> Product3/1
  Product/1 -> Sum4/1
  Sum4/1 -> Gain/1
  Trigonometric Function3/1 -> Product/2
  Gain/1 -> f_qs/1
  Gain1/1 -> f_ds/1
  Product2/1 -> Sum4/2
  Product1/1 -> Sum3/1
  Product4/1 -> Sum4/3
  Product3/1 -> Sum3/2
  Sum2/1 -> Gain2/1
  Trigonometric Function4/1 -> Product2/1
  Trigonometric Function/1 -> Product1/2
  Sum3/1 -> Gain1/1

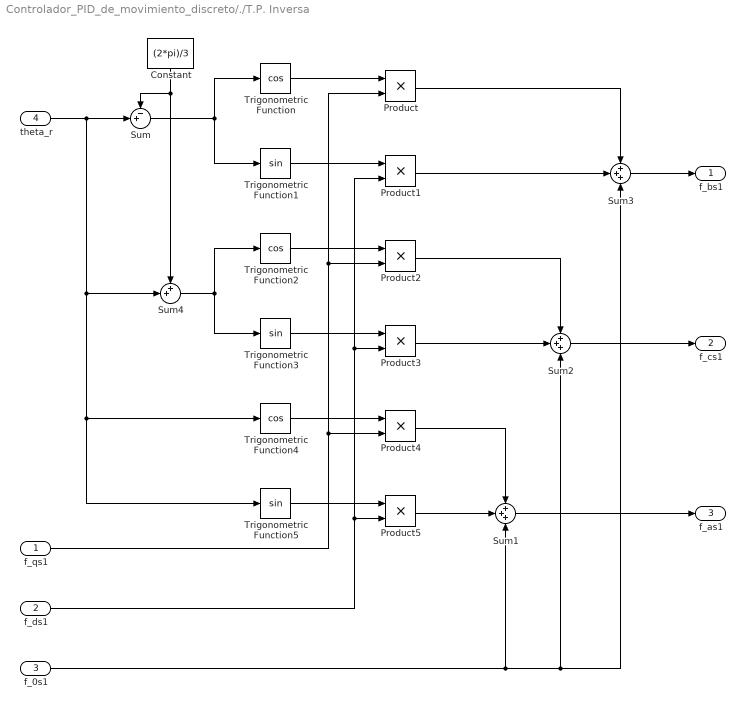
== system Controlador_PID_de_movimiento_discreto/./T.P. Inversa ==
  f_qs1 : Inport
  f_ds1 : Inport  Port=2
  f_0s1 : Inport  Port=3
  theta_r : Inport  Port=4
  Constant : Constant  Value=(2*pi)/3
  Product{,1..5} (6 alike) : Product
  Sum : Sum  Inputs=-+|
  Sum1 : Sum  Inputs=+++
  Sum2 : Sum  Inputs=+++
  Sum3 : Sum  Inputs=+++
  Sum4 : Sum  Inputs=++|
  Trigonometric Function : Trigonometry  Operator=cos
  Trigonometric Function1 : Trigonometry
  Trigonometric Function2 : Trigonometry  Operator=cos
  Trigonometric Function3 : Trigonometry
  Trigonometric Function4 : Trigonometry  Operator=cos
  Trigonometric Function5 : Trigonometry
  f_bs1 : Outport
  f_cs1 : Outport  Port=2
  f_as1 : Outport  Port=3
  wires:
  theta_r/1 -> Sum4/2, Trigonometric Function5/1, Trigonometric Function4/1, Sum/2
  Trigonometric Function3/1 -> Product3/1
  Product4/1 -> Sum1/1
  Product1/1 -> Sum3/2
  Trigonometric Function2/1 -> Product2/1
  Product2/1 -> Sum2/1
  f_0s1/1 -> Sum3/3, Sum2/3, Sum1/3
  f_qs1/1 -> Product4/2, Product2/2, Product/2
  Product5/1 -> Sum1/2
  Trigonometric Function1/1 -> Product1/1
  Sum/1 -> Trigonometric Function1/1, Trigonometric Function/1
  Trigonometric Function5/1 -> Product5/1
  Sum4/1 -> Trigonometric Function3/1, Trigonometric Function2/1
  Product/1 -> Sum3/1
  Product3/1 -> Sum2/2
  Trigonometric Function/1 -> Product/1
  Sum2/1 -> f_cs1/1
  Sum3/1 -> f_bs1/1
  f_ds1/1 -> Product5/2, Product3/2, Product1/2
  Trigonometric Function4/1 -> Product4/1
  Sum1/1 -> f_as1/1
  Constant/1 -> Sum4/1, Sum/1

== system Controlador_PID_de_movimiento_discreto/.1/Subsistema Electromagnético ==
  R_s : Inport
  v_qs : Inport  Port=2
  v_ds : Inport  Port=3
  v_0s : Inport  Port=4
  omega_m : Inport  Port=5
  corriente_i_0s : Subsystem
  corriente_i_ds : Subsystem
  corriente_i_qs : Subsystem
  torque_T_m : Subsystem
  i_0s : Outport
  i_ds : Outport  Port=2
  i_qs : Outport  Port=3
  T_m : Outport  Port=4
  wires:
  R_s/1 -> corriente_i_qs/3(R_s), corriente_i_ds/4(R_s), corriente_i_0s/2(R_s)
  corriente_i_0s/1(i_0s) -> i_0s/1
  corriente_i_qs/1(i_qs) -> i_qs/1, torque_T_m/2(i_qs), corriente_i_ds/2(i_qs)
  corriente_i_ds/1(i_ds) -> corriente_i_qs/4(i_ds), torque_T_m/1(i_ds), i_ds/1
  v_0s/1 -> corriente_i_0s/1(v_0s)
  v_ds/1 -> corriente_i_ds/1(v_ds)
  omega_m/1 -> corriente_i_qs/1(omega_m), corriente_i_ds/3(omega_m)
  v_qs/1 -> corriente_i_qs/2(v_qs)
  torque_T_m/1(T_m) -> T_m/1

== system Controlador_PID_de_movimiento_discreto/.1/Subsistema Mecánico ==
  T_m : Inport
  T_ld : Inport  Port=2
  Constant : Constant  Value=g
  Gain : Gain  Gain=1/J_eq
  Gain1 : Gain  Gain=b_eq
  Gain2 : Gain  Gain=1/r
  Gain3 : Gain  Gain=k_l
  Gain4 : Gain  Gain=1/r
  Product : Product
  Sum : Sum  Inputs=-+-
  Sum1 : Sum
  Trigonometric Function : Trigonometry
  "omega_m(0) = 0\t" : Integrator
  theta_m(0) = 0 : Integrator
  omega_m : Outport
  theta_m : Outport  Port=2
  wires:
  Product/1 -> Sum1/2
  Constant/1 -> Product/1
  T_m/1 -> Sum/2
  Gain3/1 -> Product/2
  T_ld/1 -> Sum1/1
  Gain1/1 -> Sum/3
  Gain4/1 -> Sum/1
  Sum1/1 -> Gain4/1  "T_l"
  theta_m(0) = 0/1 -> Gain2/1, theta_m/1  "theta_m(t)"
  Trigonometric Function/1 -> Gain3/1
  Sum/1 -> Gain/1
  Gain2/1 -> Trigonometric Function/1
  "omega_m(0) = 0\t"/1 -> theta_m(0) = 0/1, omega_m/1, Gain1/1  "omega_m(t)"
  Gain/1 -> "omega_m(0) = 0\t"/1  "domega_m(t)/dt"

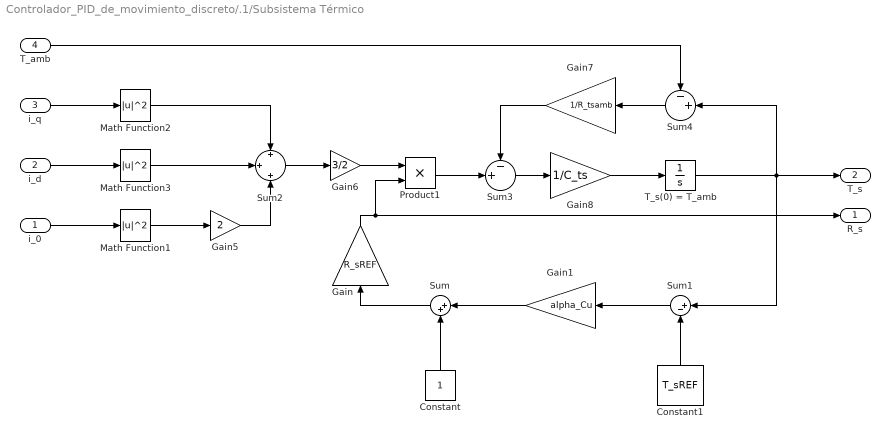
== system Controlador_PID_de_movimiento_discreto/.1/Subsistema Térmico ==
  i_0 : Inport
  i_d : Inport  Port=2
  i_q : Inport  Port=3
  T_amb : Inport  Port=4
  Constant : Constant
  Constant1 : Constant  Value=T_sREF
  Gain : Gain  Gain=R_sREF
  Gain1 : Gain  Gain=alpha_Cu
  Gain5 : Gain  Gain=2
  Gain6 : Gain  Gain=3/2
  Gain7 : Gain  Gain=1/R_tsamb
  Gain8 : Gain  Gain=1/C_ts
  Math Function1 : Math  Operator=magnitude^2  OutputSignalType=real
  Math Function2 : Math  Operator=magnitude^2  OutputSignalType=real
  Math Function3 : Math  Operator=magnitude^2  OutputSignalType=real
  Product1 : Product
  Sum : Sum  Inputs=|++
  Sum1 : Sum  Inputs=|+-
  Sum2 : Sum  Inputs=+|+|+
  Sum3 : Sum  Inputs=-+|
  Sum4 : Sum  Inputs=-+|
  T_s(0) = T_amb : Integrator  InitialCondition=T_amb
  R_s : Outport
  T_s : Outport  Port=2
  wires:
  i_q/1 -> Math Function2/1
  i_d/1 -> Math Function3/1
  i_0/1 -> Math Function1/1
  Gain1/1 -> Sum/1
  Gain8/1 -> T_s(0) = T_amb/1
  Sum3/1 -> Gain8/1
  Constant/1 -> Sum/2
  Product1/1 -> Sum3/2
  Sum/1 -> Gain/1
  T_amb/1 -> Sum4/1
  Math Function1/1 -> Gain5/1
  Sum4/1 -> Gain7/1
  T_s(0) = T_amb/1 -> Sum1/1, Sum4/2, T_s/1
  Sum2/1 -> Gain6/1
  Sum1/1 -> Gain1/1
  Gain6/1 -> Product1/1
  Constant1/1 -> Sum1/2
  Gain5/1 -> Sum2/3
  Gain7/1 -> Sum3/1
  Math Function2/1 -> Sum2/1
  Math Function3/1 -> Sum2/2
  Gain/1 -> R_s/1, Product1/2

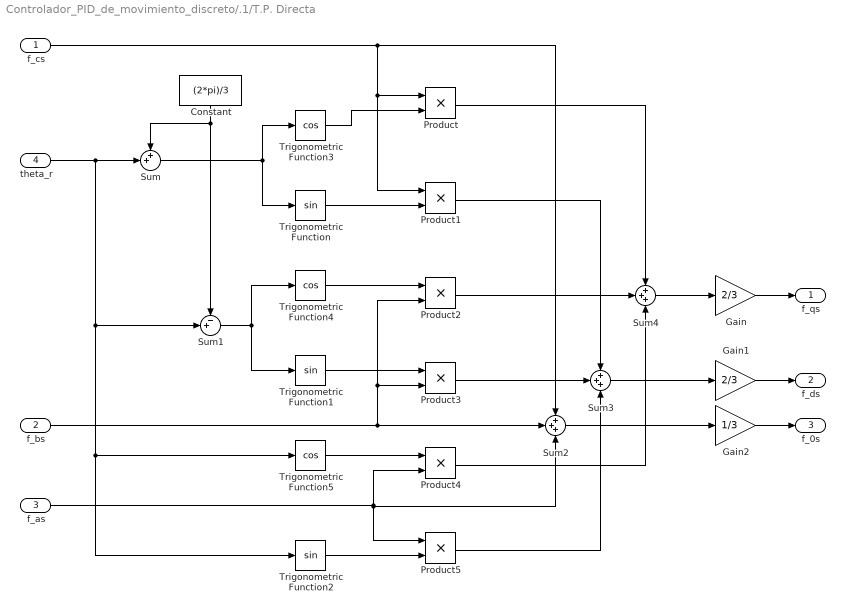
== system Controlador_PID_de_movimiento_discreto/.1/T.P. Directa ==
  f_cs : Inport
  f_bs : Inport  Port=2
  f_as : Inport  Port=3
  theta_r : Inport  Port=4
  Constant : Constant  Value=(2*pi)/3
  Gain : Gain  Gain=2/3
  Gain1 : Gain  Gain=2/3
  Gain2 : Gain  Gain=1/3
  Product{,1..5} (6 alike) : Product
  Sum : Sum  Inputs=++|
  Sum1 : Sum  Inputs=-+|
  Sum2 : Sum  Inputs=+++
  Sum3 : Sum  Inputs=+++
  Sum4 : Sum  Inputs=+++
  Trigonometric Function : Trigonometry
  Trigonometric Function1 : Trigonometry
  Trigonometric Function2 : Trigonometry
  Trigonometric Function3 : Trigonometry  Operator=cos
  Trigonometric Function4 : Trigonometry  Operator=cos
  Trigonometric Function5 : Trigonometry  Operator=cos
  f_qs : Outport
  f_ds : Outport  Port=2
  f_0s : Outport  Port=3
  wires:
  Product5/1 -> Sum3/3
  theta_r/1 -> Sum1/2, Trigonometric Function2/1, Trigonometric Function5/1, Sum/2
  f_bs/1 -> Product2/2, Product3/2, Sum2/2
  f_cs/1 -> Product/1, Product1/1, Sum2/1
  Trigonometric Function5/1 -> Product4/1
  Sum1/1 -> Trigonometric Function1/1, Trigonometric Function4/1
  Constant/1 -> Sum/1, Sum1/1
  Sum/1 -> Trigonometric Function3/1, Trigonometric Function/1
  f_as/1 -> Sum2/3, Product5/1, Product4/2
  Gain2/1 -> f_0s/1
  Trigonometric Function2/1 -> Product5/2
  Trigonometric Function1/1 -> Product3/1
  Product/1 -> Sum4/1
  Sum4/1 -> Gain/1
  Trigonometric Function3/1 -> Product/2
  Gain/1 -> f_qs/1
  Gain1/1 -> f_ds/1
  Product2/1 -> Sum4/2
  Product1/1 -> Sum3/1
  Product4/1 -> Sum4/3
  Product3/1 -> Sum3/2
  Sum2/1 -> Gain2/1
  Trigonometric Function4/1 -> Product2/1
  Trigonometric Function/1 -> Product1/2
  Sum3/1 -> Gain1/1

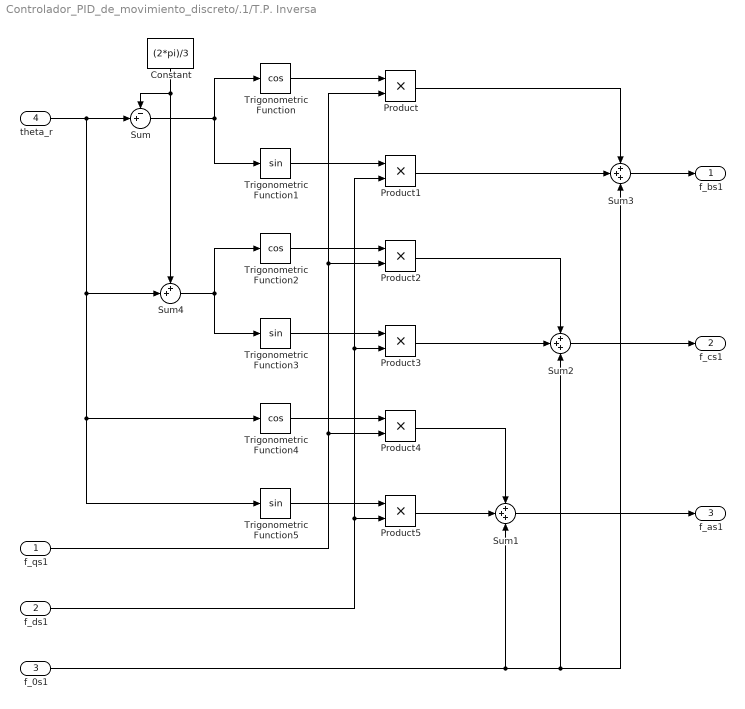
== system Controlador_PID_de_movimiento_discreto/.1/T.P. Inversa ==
  f_qs1 : Inport
  f_ds1 : Inport  Port=2
  f_0s1 : Inport  Port=3
  theta_r : Inport  Port=4
  Constant : Constant  Value=(2*pi)/3
  Product{,1..5} (6 alike) : Product
  Sum : Sum  Inputs=-+|
  Sum1 : Sum  Inputs=+++
  Sum2 : Sum  Inputs=+++
  Sum3 : Sum  Inputs=+++
  Sum4 : Sum  Inputs=++|
  Trigonometric Function : Trigonometry  Operator=cos
  Trigonometric Function1 : Trigonometry
  Trigonometric Function2 : Trigonometry  Operator=cos
  Trigonometric Function3 : Trigonometry
  Trigonometric Function4 : Trigonometry  Operator=cos
  Trigonometric Function5 : Trigonometry
  f_bs1 : Outport
  f_cs1 : Outport  Port=2
  f_as1 : Outport  Port=3
  wires:
  theta_r/1 -> Sum4/2, Trigonometric Function5/1, Trigonometric Function4/1, Sum/2
  Trigonometric Function3/1 -> Product3/1
  Product4/1 -> Sum1/1
  Product1/1 -> Sum3/2
  Trigonometric Function2/1 -> Product2/1
  Product2/1 -> Sum2/1
  f_0s1/1 -> Sum3/3, Sum2/3, Sum1/3
  f_qs1/1 -> Product4/2, Product2/2, Product/2
  Product5/1 -> Sum1/2
  Trigonometric Function1/1 -> Product1/1
  Sum/1 -> Trigonometric Function1/1, Trigonometric Function/1
  Trigonometric Function5/1 -> Product5/1
  Sum4/1 -> Trigonometric Function3/1, Trigonometric Function2/1
  Product/1 -> Sum3/1
  Product3/1 -> Sum2/2
  Trigonometric Function/1 -> Product/1
  Sum2/1 -> f_cs1/1
  Sum3/1 -> f_bs1/1
  f_ds1/1 -> Product5/2, Product3/2, Product1/2
  Trigonometric Function4/1 -> Product4/1
  Sum1/1 -> f_as1/1
  Constant/1 -> Sum4/1, Sum/1

== system Controlador_PID_de_movimiento_discreto/Controlador PID de movimiento discreto1/Integrador discreto ==
  u : Inport
  Gain : Gain  Gain=Ts/2
  Sum : Sum  Inputs=|++
  Sum1 : Sum  Inputs=|++
  Unit Delay : UnitDelay  SampleTime=Ts  HasFrameUpgradeWarning=on
  Unit Delay1 : UnitDelay  SampleTime=Ts  HasFrameUpgradeWarning=on
  y : Outport
  wires:
  Unit Delay/1 -> Sum1/2
  Gain/1 -> Sum1/1
  Unit Delay1/1 -> Sum/2
  u/1 -> Unit Delay1/1, Sum/1
  Sum1/1 -> y/1, Unit Delay/1
  Sum/1 -> Gain/1

== system Controlador_PID_de_movimiento_discreto/Controlador PID de movimiento discreto1/Integrador discreto1 ==
  u : Inport
  Gain : Gain  Gain=Ts/2
  Sum : Sum  Inputs=|++
  Sum1 : Sum  Inputs=|++
  Unit Delay : UnitDelay  SampleTime=Ts  HasFrameUpgradeWarning=on
  Unit Delay1 : UnitDelay  SampleTime=Ts  HasFrameUpgradeWarning=on
  y : Outport
  wires:
  Sum/1 -> Gain/1
  Sum1/1 -> Unit Delay/1, y/1
  u/1 -> Sum/1, Unit Delay1/1
  Unit Delay1/1 -> Sum/2
  Gain/1 -> Sum1/1
  Unit Delay/1 -> Sum1/2
